simulink model "c00019M_harness"  (R2018a)
settings: Solver=ode3  StartTime=0.0  StopTime=10.0  RelTol=1e-3  EnableMultiTasking=on
undefined symbols (not defined in the file): b, DiscIntNeverNeededParam, J, K, L, PosMinimaW4, R, sigbuilder_block
(part 7 of 43)

== system c00019M_harness/M063 ==
  DW1 : Inport  OutMin=0  OutMax=4  OutDataTypeStr=int8
  P1W2 : Inport  Port=2  OutMin=0  OutMax=4  OutDataTypeStr=int8
  P3W4 : Inport  Port=3  OutMin=0  OutMax=4  OutDataTypeStr=int8
  O1 : Inport  Port=4  OutDataTypeStr=boolean
  O2 : Inport  Port=5  OutDataTypeStr=boolean
  O4 : Inport  Port=6  OutDataTypeStr=boolean
  LD : Inport  Port=7  OutDataTypeStr=boolean
  CW1C : Inport  Port=8  OutMin=0  OutMax=4  OutDataTypeStr=int8
  CW2C : Inport  Port=9  OutMin=0  OutMax=4  OutDataTypeStr=int8
  CW4C : Inport  Port=10  OutMin=0  OutMax=4  OutDataTypeStr=int8
  Cyber : Subsystem
  M : Memory
  M1 : Memory
  M3 : Memory
  Physical : Subsystem
  S1 : Subsystem
  S2 : Subsystem
  S4 : Subsystem
  W1Pos : Outport
  W2Pos : Outport  Port=2
  W4Pos : Outport  Port=3
  wires:
  Cyber/3(W4) -> Physical/3(InW4)
  Physical/3(W4) -> S4/1(PhyMeasure), W4Pos/1
  P3W4/1 -> Cyber/6(P3W4)
  S2/1(SensorOut) -> M1/1
  Physical/2(W2) -> S2/1(PhyMeasure), W2Pos/1
  DW1/1 -> Cyber/4(DW1)
  M/1 -> Cyber/1(PosW1)
  M1/1 -> Cyber/2(PosW2)
  S4/1(SensorOut) -> M3/1
  CW1C/1 -> Cyber/11(CW1C)
  P1W2/1 -> Cyber/5(P1W2)
  Cyber/2(W2) -> Physical/2(InW2)
  Cyber/1(W1) -> Physical/1(InW1)
  O1/1 -> Cyber/7(OW1)
  LD/1 -> Cyber/10(LD)
  O2/1 -> Cyber/8(OW2)
  O4/1 -> Cyber/9(OW4)
  Physical/1(W1) -> S1/1(PhyMeasure), W1Pos/1
  CW4C/1 -> Cyber/13(CW4C)
  CW2C/1 -> Cyber/12(CW2C)
  S1/1(SensorOut) -> M/1
  M3/1 -> Cyber/3(PosW4)

== system c00019M_harness/M064 ==
  DW1 : Inport  OutMin=0  OutMax=4  OutDataTypeStr=int8
  P1W2 : Inport  Port=2  OutMin=0  OutMax=4  OutDataTypeStr=int8
  P3W4 : Inport  Port=3  OutMin=0  OutMax=4  OutDataTypeStr=int8
  O1 : Inport  Port=4  OutDataTypeStr=boolean
  O2 : Inport  Port=5  OutDataTypeStr=boolean
  O4 : Inport  Port=6  OutDataTypeStr=boolean
  LD : Inport  Port=7  OutDataTypeStr=boolean
  CW1C : Inport  Port=8  OutMin=0  OutMax=4  OutDataTypeStr=int8
  CW2C : Inport  Port=9  OutMin=0  OutMax=4  OutDataTypeStr=int8
  CW4C : Inport  Port=10  OutMin=0  OutMax=4  OutDataTypeStr=int8
  Cyber : Subsystem
  M : Memory
  M1 : Memory
  M3 : Memory
  Physical : Subsystem
  S1 : Subsystem
  S2 : Subsystem
  S4 : Subsystem
  W1Pos : Outport
  W2Pos : Outport  Port=2
  W4Pos : Outport  Port=3
  wires:
  Cyber/3(W4) -> Physical/3(InW4)
  Physical/3(W4) -> S4/1(PhyMeasure), W4Pos/1
  P3W4/1 -> Cyber/6(P3W4)
  S2/1(SensorOut) -> M1/1
  Physical/2(W2) -> S2/1(PhyMeasure), W2Pos/1
  DW1/1 -> Cyber/4(DW1)
  M/1 -> Cyber/1(PosW1)
  M1/1 -> Cyber/2(PosW2)
  S4/1(SensorOut) -> M3/1
  CW1C/1 -> Cyber/11(CW1C)
  P1W2/1 -> Cyber/5(P1W2)
  Cyber/2(W2) -> Physical/2(InW2)
  Cyber/1(W1) -> Physical/1(InW1)
  O1/1 -> Cyber/7(OW1)
  LD/1 -> Cyber/10(LD)
  O2/1 -> Cyber/8(OW2)
  O4/1 -> Cyber/9(OW4)
  Physical/1(W1) -> S1/1(PhyMeasure), W1Pos/1
  CW4C/1 -> Cyber/13(CW4C)
  CW2C/1 -> Cyber/12(CW2C)
  S1/1(SensorOut) -> M/1
  M3/1 -> Cyber/3(PosW4)

== system c00019M_harness/M066 ==
  DW1 : Inport  OutMin=0  OutMax=4  OutDataTypeStr=int8
  P1W2 : Inport  Port=2  OutMin=0  OutMax=4  OutDataTypeStr=int8
  P3W4 : Inport  Port=3  OutMin=0  OutMax=4  OutDataTypeStr=int8
  O1 : Inport  Port=4  OutDataTypeStr=boolean
  O2 : Inport  Port=5  OutDataTypeStr=boolean
  O4 : Inport  Port=6  OutDataTypeStr=boolean
  LD : Inport  Port=7  OutDataTypeStr=boolean
  CW1C : Inport  Port=8  OutMin=0  OutMax=4  OutDataTypeStr=int8
  CW2C : Inport  Port=9  OutMin=0  OutMax=4  OutDataTypeStr=int8
  CW4C : Inport  Port=10  OutMin=0  OutMax=4  OutDataTypeStr=int8
  Cyber : Subsystem
  M : Memory
  M1 : Memory
  M3 : Memory
  Physical : Subsystem
  S1 : Subsystem
  S2 : Subsystem
  S4 : Subsystem
  W1Pos : Outport
  W2Pos : Outport  Port=2
  W4Pos : Outport  Port=3
  wires:
  Cyber/3(W4) -> Physical/3(InW4)
  Physical/3(W4) -> S4/1(PhyMeasure), W4Pos/1
  P3W4/1 -> Cyber/6(P3W4)
  S2/1(SensorOut) -> M1/1
  Physical/2(W2) -> S2/1(PhyMeasure), W2Pos/1
  DW1/1 -> Cyber/4(DW1)
  M/1 -> Cyber/1(PosW1)
  M1/1 -> Cyber/2(PosW2)
  S4/1(SensorOut) -> M3/1
  CW1C/1 -> Cyber/11(CW1C)
  P1W2/1 -> Cyber/5(P1W2)
  Cyber/2(W2) -> Physical/2(InW2)
  Cyber/1(W1) -> Physical/1(InW1)
  O1/1 -> Cyber/7(OW1)
  LD/1 -> Cyber/10(LD)
  O2/1 -> Cyber/8(OW2)
  O4/1 -> Cyber/9(OW4)
  Physical/1(W1) -> S1/1(PhyMeasure), W1Pos/1
  CW4C/1 -> Cyber/13(CW4C)
  CW2C/1 -> Cyber/12(CW2C)
  S1/1(SensorOut) -> M/1
  M3/1 -> Cyber/3(PosW4)

== system c00019M_harness/M067 ==
  DW1 : Inport  OutMin=0  OutMax=4  OutDataTypeStr=int8
  P1W2 : Inport  Port=2  OutMin=0  OutMax=4  OutDataTypeStr=int8
  P3W4 : Inport  Port=3  OutMin=0  OutMax=4  OutDataTypeStr=int8
  O1 : Inport  Port=4  OutDataTypeStr=boolean
  O2 : Inport  Port=5  OutDataTypeStr=boolean
  O4 : Inport  Port=6  OutDataTypeStr=boolean
  LD : Inport  Port=7  OutDataTypeStr=boolean
  CW1C : Inport  Port=8  OutMin=0  OutMax=4  OutDataTypeStr=int8
  CW2C : Inport  Port=9  OutMin=0  OutMax=4  OutDataTypeStr=int8
  CW4C : Inport  Port=10  OutMin=0  OutMax=4  OutDataTypeStr=int8
  Cyber : Subsystem
  M : Memory
  M1 : Memory
  M3 : Memory
  Physical : Subsystem
  S1 : Subsystem
  S2 : Subsystem
  S4 : Subsystem
  W1Pos : Outport
  W2Pos : Outport  Port=2
  W4Pos : Outport  Port=3
  wires:
  Cyber/3(W4) -> Physical/3(InW4)
  Physical/3(W4) -> S4/1(PhyMeasure), W4Pos/1
  P3W4/1 -> Cyber/6(P3W4)
  S2/1(SensorOut) -> M1/1
  Physical/2(W2) -> S2/1(PhyMeasure), W2Pos/1
  DW1/1 -> Cyber/4(DW1)
  M/1 -> Cyber/1(PosW1)
  M1/1 -> Cyber/2(PosW2)
  S4/1(SensorOut) -> M3/1
  CW1C/1 -> Cyber/11(CW1C)
  P1W2/1 -> Cyber/5(P1W2)
  Cyber/2(W2) -> Physical/2(InW2)
  Cyber/1(W1) -> Physical/1(InW1)
  O1/1 -> Cyber/7(OW1)
  LD/1 -> Cyber/10(LD)
  O2/1 -> Cyber/8(OW2)
  O4/1 -> Cyber/9(OW4)
  Physical/1(W1) -> S1/1(PhyMeasure), W1Pos/1
  CW4C/1 -> Cyber/13(CW4C)
  CW2C/1 -> Cyber/12(CW2C)
  S1/1(SensorOut) -> M/1
  M3/1 -> Cyber/3(PosW4)

== system c00019M_harness/M068 ==
  DW1 : Inport  OutMin=0  OutMax=4  OutDataTypeStr=int8
  P1W2 : Inport  Port=2  OutMin=0  OutMax=4  OutDataTypeStr=int8
  P3W4 : Inport  Port=3  OutMin=0  OutMax=4  OutDataTypeStr=int8
  O1 : Inport  Port=4  OutDataTypeStr=boolean
  O2 : Inport  Port=5  OutDataTypeStr=boolean
  O4 : Inport  Port=6  OutDataTypeStr=boolean
  LD : Inport  Port=7  OutDataTypeStr=boolean
  CW1C : Inport  Port=8  OutMin=0  OutMax=4  OutDataTypeStr=int8
  CW2C : Inport  Port=9  OutMin=0  OutMax=4  OutDataTypeStr=int8
  CW4C : Inport  Port=10  OutMin=0  OutMax=4  OutDataTypeStr=int8
  Cyber : Subsystem
  M : Memory
  M1 : Memory
  M3 : Memory
  Physical : Subsystem
  S1 : Subsystem
  S2 : Subsystem
  S4 : Subsystem
  W1Pos : Outport
  W2Pos : Outport  Port=2
  W4Pos : Outport  Port=3
  wires:
  Cyber/3(W4) -> Physical/3(InW4)
  Physical/3(W4) -> S4/1(PhyMeasure), W4Pos/1
  P3W4/1 -> Cyber/6(P3W4)
  S2/1(SensorOut) -> M1/1
  Physical/2(W2) -> S2/1(PhyMeasure), W2Pos/1
  DW1/1 -> Cyber/4(DW1)
  M/1 -> Cyber/1(PosW1)
  M1/1 -> Cyber/2(PosW2)
  S4/1(SensorOut) -> M3/1
  CW1C/1 -> Cyber/11(CW1C)
  P1W2/1 -> Cyber/5(P1W2)
  Cyber/2(W2) -> Physical/2(InW2)
  Cyber/1(W1) -> Physical/1(InW1)
  O1/1 -> Cyber/7(OW1)
  LD/1 -> Cyber/10(LD)
  O2/1 -> Cyber/8(OW2)
  O4/1 -> Cyber/9(OW4)
  Physical/1(W1) -> S1/1(PhyMeasure), W1Pos/1
  CW4C/1 -> Cyber/13(CW4C)
  CW2C/1 -> Cyber/12(CW2C)
  S1/1(SensorOut) -> M/1
  M3/1 -> Cyber/3(PosW4)

== system c00019M_harness/M070 ==
  DW1 : Inport  OutMin=0  OutMax=4  OutDataTypeStr=int8
  P1W2 : Inport  Port=2  OutMin=0  OutMax=4  OutDataTypeStr=int8
  P3W4 : Inport  Port=3  OutMin=0  OutMax=4  OutDataTypeStr=int8
  O1 : Inport  Port=4  OutDataTypeStr=boolean
  O2 : Inport  Port=5  OutDataTypeStr=boolean
  O4 : Inport  Port=6  OutDataTypeStr=boolean
  LD : Inport  Port=7  OutDataTypeStr=boolean
  CW1C : Inport  Port=8  OutMin=0  OutMax=4  OutDataTypeStr=int8
  CW2C : Inport  Port=9  OutMin=0  OutMax=4  OutDataTypeStr=int8
  CW4C : Inport  Port=10  OutMin=0  OutMax=4  OutDataTypeStr=int8
  Cyber : Subsystem
  M : Memory
  M1 : Memory
  M3 : Memory
  Physical : Subsystem
  S1 : Subsystem
  S2 : Subsystem
  S4 : Subsystem
  W1Pos : Outport
  W2Pos : Outport  Port=2
  W4Pos : Outport  Port=3
  wires:
  Cyber/3(W4) -> Physical/3(InW4)
  Physical/3(W4) -> S4/1(PhyMeasure), W4Pos/1
  P3W4/1 -> Cyber/6(P3W4)
  S2/1(SensorOut) -> M1/1
  Physical/2(W2) -> S2/1(PhyMeasure), W2Pos/1
  DW1/1 -> Cyber/4(DW1)
  M/1 -> Cyber/1(PosW1)
  M1/1 -> Cyber/2(PosW2)
  S4/1(SensorOut) -> M3/1
  CW1C/1 -> Cyber/11(CW1C)
  P1W2/1 -> Cyber/5(P1W2)
  Cyber/2(W2) -> Physical/2(InW2)
  Cyber/1(W1) -> Physical/1(InW1)
  O1/1 -> Cyber/7(OW1)
  LD/1 -> Cyber/10(LD)
  O2/1 -> Cyber/8(OW2)
  O4/1 -> Cyber/9(OW4)
  Physical/1(W1) -> S1/1(PhyMeasure), W1Pos/1
  CW4C/1 -> Cyber/13(CW4C)
  CW2C/1 -> Cyber/12(CW2C)
  S1/1(SensorOut) -> M/1
  M3/1 -> Cyber/3(PosW4)

== system c00019M_harness/M071 ==
  DW1 : Inport  OutMin=0  OutMax=4  OutDataTypeStr=int8
  P1W2 : Inport  Port=2  OutMin=0  OutMax=4  OutDataTypeStr=int8
  P3W4 : Inport  Port=3  OutMin=0  OutMax=4  OutDataTypeStr=int8
  O1 : Inport  Port=4  OutDataTypeStr=boolean
  O2 : Inport  Port=5  OutDataTypeStr=boolean
  O4 : Inport  Port=6  OutDataTypeStr=boolean
  LD : Inport  Port=7  OutDataTypeStr=boolean
  CW1C : Inport  Port=8  OutMin=0  OutMax=4  OutDataTypeStr=int8
  CW2C : Inport  Port=9  OutMin=0  OutMax=4  OutDataTypeStr=int8
  CW4C : Inport  Port=10  OutMin=0  OutMax=4  OutDataTypeStr=int8
  Cyber : Subsystem
  M : Memory
  M1 : Memory
  M3 : Memory
  Physical : Subsystem
  S1 : Subsystem
  S2 : Subsystem
  S4 : Subsystem
  W1Pos : Outport
  W2Pos : Outport  Port=2
  W4Pos : Outport  Port=3
  wires:
  Cyber/3(W4) -> Physical/3(InW4)
  Physical/3(W4) -> S4/1(PhyMeasure), W4Pos/1
  P3W4/1 -> Cyber/6(P3W4)
  S2/1(SensorOut) -> M1/1
  Physical/2(W2) -> S2/1(PhyMeasure), W2Pos/1
  DW1/1 -> Cyber/4(DW1)
  M/1 -> Cyber/1(PosW1)
  M1/1 -> Cyber/2(PosW2)
  S4/1(SensorOut) -> M3/1
  CW1C/1 -> Cyber/11(CW1C)
  P1W2/1 -> Cyber/5(P1W2)
  Cyber/2(W2) -> Physical/2(InW2)
  Cyber/1(W1) -> Physical/1(InW1)
  O1/1 -> Cyber/7(OW1)
  LD/1 -> Cyber/10(LD)
  O2/1 -> Cyber/8(OW2)
  O4/1 -> Cyber/9(OW4)
  Physical/1(W1) -> S1/1(PhyMeasure), W1Pos/1
  CW4C/1 -> Cyber/13(CW4C)
  CW2C/1 -> Cyber/12(CW2C)
  S1/1(SensorOut) -> M/1
  M3/1 -> Cyber/3(PosW4)

== system c00019M_harness/M072 ==
  DW1 : Inport  OutMin=0  OutMax=4  OutDataTypeStr=int8
  P1W2 : Inport  Port=2  OutMin=0  OutMax=4  OutDataTypeStr=int8
  P3W4 : Inport  Port=3  OutMin=0  OutMax=4  OutDataTypeStr=int8
  O1 : Inport  Port=4  OutDataTypeStr=boolean
  O2 : Inport  Port=5  OutDataTypeStr=boolean
  O4 : Inport  Port=6  OutDataTypeStr=boolean
  LD : Inport  Port=7  OutDataTypeStr=boolean
  CW1C : Inport  Port=8  OutMin=0  OutMax=4  OutDataTypeStr=int8
  CW2C : Inport  Port=9  OutMin=0  OutMax=4  OutDataTypeStr=int8
  CW4C : Inport  Port=10  OutMin=0  OutMax=4  OutDataTypeStr=int8
  Cyber : Subsystem
  M : Memory
  M1 : Memory
  M3 : Memory
  Physical : Subsystem
  S1 : Subsystem
  S2 : Subsystem
  S4 : Subsystem
  W1Pos : Outport
  W2Pos : Outport  Port=2
  W4Pos : Outport  Port=3
  wires:
  Cyber/3(W4) -> Physical/3(InW4)
  Physical/3(W4) -> S4/1(PhyMeasure), W4Pos/1
  P3W4/1 -> Cyber/6(P3W4)
  S2/1(SensorOut) -> M1/1
  Physical/2(W2) -> S2/1(PhyMeasure), W2Pos/1
  DW1/1 -> Cyber/4(DW1)
  M/1 -> Cyber/1(PosW1)
  M1/1 -> Cyber/2(PosW2)
  S4/1(SensorOut) -> M3/1
  CW1C/1 -> Cyber/11(CW1C)
  P1W2/1 -> Cyber/5(P1W2)
  Cyber/2(W2) -> Physical/2(InW2)
  Cyber/1(W1) -> Physical/1(InW1)
  O1/1 -> Cyber/7(OW1)
  LD/1 -> Cyber/10(LD)
  O2/1 -> Cyber/8(OW2)
  O4/1 -> Cyber/9(OW4)
  Physical/1(W1) -> S1/1(PhyMeasure), W1Pos/1
  CW4C/1 -> Cyber/13(CW4C)
  CW2C/1 -> Cyber/12(CW2C)
  S1/1(SensorOut) -> M/1
  M3/1 -> Cyber/3(PosW4)

== system c00019M_harness/M074 ==
  DW1 : Inport  OutMin=0  OutMax=4  OutDataTypeStr=int8
  P1W2 : Inport  Port=2  OutMin=0  OutMax=4  OutDataTypeStr=int8
  P3W4 : Inport  Port=3  OutMin=0  OutMax=4  OutDataTypeStr=int8
  O1 : Inport  Port=4  OutDataTypeStr=boolean
  O2 : Inport  Port=5  OutDataTypeStr=boolean
  O4 : Inport  Port=6  OutDataTypeStr=boolean
  LD : Inport  Port=7  OutDataTypeStr=boolean
  CW1C : Inport  Port=8  OutMin=0  OutMax=4  OutDataTypeStr=int8
  CW2C : Inport  Port=9  OutMin=0  OutMax=4  OutDataTypeStr=int8
  CW4C : Inport  Port=10  OutMin=0  OutMax=4  OutDataTypeStr=int8
  Cyber : Subsystem
  M : Memory
  M1 : Memory
  M3 : Memory
  Physical : Subsystem
  S1 : Subsystem
  S2 : Subsystem
  S4 : Subsystem
  W1Pos : Outport
  W2Pos : Outport  Port=2
  W4Pos : Outport  Port=3
  wires:
  Cyber/3(W4) -> Physical/3(InW4)
  Physical/3(W4) -> S4/1(PhyMeasure), W4Pos/1
  P3W4/1 -> Cyber/6(P3W4)
  S2/1(SensorOut) -> M1/1
  Physical/2(W2) -> S2/1(PhyMeasure), W2Pos/1
  DW1/1 -> Cyber/4(DW1)
  M/1 -> Cyber/1(PosW1)
  M1/1 -> Cyber/2(PosW2)
  S4/1(SensorOut) -> M3/1
  CW1C/1 -> Cyber/11(CW1C)
  P1W2/1 -> Cyber/5(P1W2)
  Cyber/2(W2) -> Physical/2(InW2)
  Cyber/1(W1) -> Physical/1(InW1)
  O1/1 -> Cyber/7(OW1)
  LD/1 -> Cyber/10(LD)
  O2/1 -> Cyber/8(OW2)
  O4/1 -> Cyber/9(OW4)
  Physical/1(W1) -> S1/1(PhyMeasure), W1Pos/1
  CW4C/1 -> Cyber/13(CW4C)
  CW2C/1 -> Cyber/12(CW2C)
  S1/1(SensorOut) -> M/1
  M3/1 -> Cyber/3(PosW4)

== system c00019M_harness/M075 ==
  DW1 : Inport  OutMin=0  OutMax=4  OutDataTypeStr=int8
  P1W2 : Inport  Port=2  OutMin=0  OutMax=4  OutDataTypeStr=int8
  P3W4 : Inport  Port=3  OutMin=0  OutMax=4  OutDataTypeStr=int8
  O1 : Inport  Port=4  OutDataTypeStr=boolean
  O2 : Inport  Port=5  OutDataTypeStr=boolean
  O4 : Inport  Port=6  OutDataTypeStr=boolean
  LD : Inport  Port=7  OutDataTypeStr=boolean
  CW1C : Inport  Port=8  OutMin=0  OutMax=4  OutDataTypeStr=int8
  CW2C : Inport  Port=9  OutMin=0  OutMax=4  OutDataTypeStr=int8
  CW4C : Inport  Port=10  OutMin=0  OutMax=4  OutDataTypeStr=int8
  Cyber : Subsystem
  M : Memory
  M1 : Memory
  M3 : Memory
  Physical : Subsystem
  S1 : Subsystem
  S2 : Subsystem
  S4 : Subsystem
  W1Pos : Outport
  W2Pos : Outport  Port=2
  W4Pos : Outport  Port=3
  wires:
  Cyber/3(W4) -> Physical/3(InW4)
  Physical/3(W4) -> S4/1(PhyMeasure), W4Pos/1
  P3W4/1 -> Cyber/6(P3W4)
  S2/1(SensorOut) -> M1/1
  Physical/2(W2) -> S2/1(PhyMeasure), W2Pos/1
  DW1/1 -> Cyber/4(DW1)
  M/1 -> Cyber/1(PosW1)
  M1/1 -> Cyber/2(PosW2)
  S4/1(SensorOut) -> M3/1
  CW1C/1 -> Cyber/11(CW1C)
  P1W2/1 -> Cyber/5(P1W2)
  Cyber/2(W2) -> Physical/2(InW2)
  Cyber/1(W1) -> Physical/1(InW1)
  O1/1 -> Cyber/7(OW1)
  LD/1 -> Cyber/10(LD)
  O2/1 -> Cyber/8(OW2)
  O4/1 -> Cyber/9(OW4)
  Physical/1(W1) -> S1/1(PhyMeasure), W1Pos/1
  CW4C/1 -> Cyber/13(CW4C)
  CW2C/1 -> Cyber/12(CW2C)
  S1/1(SensorOut) -> M/1
  M3/1 -> Cyber/3(PosW4)

== system c00019M_harness/M076 ==
  DW1 : Inport  OutMin=0  OutMax=4  OutDataTypeStr=int8
  P1W2 : Inport  Port=2  OutMin=0  OutMax=4  OutDataTypeStr=int8
  P3W4 : Inport  Port=3  OutMin=0  OutMax=4  OutDataTypeStr=int8
  O1 : Inport  Port=4  OutDataTypeStr=boolean
  O2 : Inport  Port=5  OutDataTypeStr=boolean
  O4 : Inport  Port=6  OutDataTypeStr=boolean
  LD : Inport  Port=7  OutDataTypeStr=boolean
  CW1C : Inport  Port=8  OutMin=0  OutMax=4  OutDataTypeStr=int8
  CW2C : Inport  Port=9  OutMin=0  OutMax=4  OutDataTypeStr=int8
  CW4C : Inport  Port=10  OutMin=0  OutMax=4  OutDataTypeStr=int8
  Cyber : Subsystem
  M : Memory
  M1 : Memory
  M3 : Memory
  Physical : Subsystem
  S1 : Subsystem
  S2 : Subsystem
  S4 : Subsystem
  W1Pos : Outport
  W2Pos : Outport  Port=2
  W4Pos : Outport  Port=3
  wires:
  Cyber/3(W4) -> Physical/3(InW4)
  Physical/3(W4) -> S4/1(PhyMeasure), W4Pos/1
  P3W4/1 -> Cyber/6(P3W4)
  S2/1(SensorOut) -> M1/1
  Physical/2(W2) -> S2/1(PhyMeasure), W2Pos/1
  DW1/1 -> Cyber/4(DW1)
  M/1 -> Cyber/1(PosW1)
  M1/1 -> Cyber/2(PosW2)
  S4/1(SensorOut) -> M3/1
  CW1C/1 -> Cyber/11(CW1C)
  P1W2/1 -> Cyber/5(P1W2)
  Cyber/2(W2) -> Physical/2(InW2)
  Cyber/1(W1) -> Physical/1(InW1)
  O1/1 -> Cyber/7(OW1)
  LD/1 -> Cyber/10(LD)
  O2/1 -> Cyber/8(OW2)
  O4/1 -> Cyber/9(OW4)
  Physical/1(W1) -> S1/1(PhyMeasure), W1Pos/1
  CW4C/1 -> Cyber/13(CW4C)
  CW2C/1 -> Cyber/12(CW2C)
  S1/1(SensorOut) -> M/1
  M3/1 -> Cyber/3(PosW4)

== system c00019M_harness/M078 ==
  DW1 : Inport  OutMin=0  OutMax=4  OutDataTypeStr=int8
  P1W2 : Inport  Port=2  OutMin=0  OutMax=4  OutDataTypeStr=int8
  P3W4 : Inport  Port=3  OutMin=0  OutMax=4  OutDataTypeStr=int8
  O1 : Inport  Port=4  OutDataTypeStr=boolean
  O2 : Inport  Port=5  OutDataTypeStr=boolean
  O4 : Inport  Port=6  OutDataTypeStr=boolean
  LD : Inport  Port=7  OutDataTypeStr=boolean
  CW1C : Inport  Port=8  OutMin=0  OutMax=4  OutDataTypeStr=int8
  CW2C : Inport  Port=9  OutMin=0  OutMax=4  OutDataTypeStr=int8
  CW4C : Inport  Port=10  OutMin=0  OutMax=4  OutDataTypeStr=int8
  Cyber : Subsystem
  M : Memory
  M1 : Memory
  M3 : Memory
  Physical : Subsystem
  S1 : Subsystem
  S2 : Subsystem
  S4 : Subsystem
  W1Pos : Outport
  W2Pos : Outport  Port=2
  W4Pos : Outport  Port=3
  wires:
  Cyber/3(W4) -> Physical/3(InW4)
  Physical/3(W4) -> S4/1(PhyMeasure), W4Pos/1
  P3W4/1 -> Cyber/6(P3W4)
  S2/1(SensorOut) -> M1/1
  Physical/2(W2) -> S2/1(PhyMeasure), W2Pos/1
  DW1/1 -> Cyber/4(DW1)
  M/1 -> Cyber/1(PosW1)
  M1/1 -> Cyber/2(PosW2)
  S4/1(SensorOut) -> M3/1
  CW1C/1 -> Cyber/11(CW1C)
  P1W2/1 -> Cyber/5(P1W2)
  Cyber/2(W2) -> Physical/2(InW2)
  Cyber/1(W1) -> Physical/1(InW1)
  O1/1 -> Cyber/7(OW1)
  LD/1 -> Cyber/10(LD)
  O2/1 -> Cyber/8(OW2)
  O4/1 -> Cyber/9(OW4)
  Physical/1(W1) -> S1/1(PhyMeasure), W1Pos/1
  CW4C/1 -> Cyber/13(CW4C)
  CW2C/1 -> Cyber/12(CW2C)
  S1/1(SensorOut) -> M/1
  M3/1 -> Cyber/3(PosW4)

== system c00019M_harness/M079 ==
  DW1 : Inport  OutMin=0  OutMax=4  OutDataTypeStr=int8
  P1W2 : Inport  Port=2  OutMin=0  OutMax=4  OutDataTypeStr=int8
  P3W4 : Inport  Port=3  OutMin=0  OutMax=4  OutDataTypeStr=int8
  O1 : Inport  Port=4  OutDataTypeStr=boolean
  O2 : Inport  Port=5  OutDataTypeStr=boolean
  O4 : Inport  Port=6  OutDataTypeStr=boolean
  LD : Inport  Port=7  OutDataTypeStr=boolean
  CW1C : Inport  Port=8  OutMin=0  OutMax=4  OutDataTypeStr=int8
  CW2C : Inport  Port=9  OutMin=0  OutMax=4  OutDataTypeStr=int8
  CW4C : Inport  Port=10  OutMin=0  OutMax=4  OutDataTypeStr=int8
  Cyber : Subsystem
  M : Memory
  M1 : Memory
  M3 : Memory
  Physical : Subsystem
  S1 : Subsystem
  S2 : Subsystem
  S4 : Subsystem
  W1Pos : Outport
  W2Pos : Outport  Port=2
  W4Pos : Outport  Port=3
  wires:
  Cyber/3(W4) -> Physical/3(InW4)
  Physical/3(W4) -> S4/1(PhyMeasure), W4Pos/1
  P3W4/1 -> Cyber/6(P3W4)
  S2/1(SensorOut) -> M1/1
  Physical/2(W2) -> S2/1(PhyMeasure), W2Pos/1
  DW1/1 -> Cyber/4(DW1)
  M/1 -> Cyber/1(PosW1)
  M1/1 -> Cyber/2(PosW2)
  S4/1(SensorOut) -> M3/1
  CW1C/1 -> Cyber/11(CW1C)
  P1W2/1 -> Cyber/5(P1W2)
  Cyber/2(W2) -> Physical/2(InW2)
  Cyber/1(W1) -> Physical/1(InW1)
  O1/1 -> Cyber/7(OW1)
  LD/1 -> Cyber/10(LD)
  O2/1 -> Cyber/8(OW2)
  O4/1 -> Cyber/9(OW4)
  Physical/1(W1) -> S1/1(PhyMeasure), W1Pos/1
  CW4C/1 -> Cyber/13(CW4C)
  CW2C/1 -> Cyber/12(CW2C)
  S1/1(SensorOut) -> M/1
  M3/1 -> Cyber/3(PosW4)

== system c00019M_harness/M080 ==
  DW1 : Inport  OutMin=0  OutMax=4  OutDataTypeStr=int8
  P1W2 : Inport  Port=2  OutMin=0  OutMax=4  OutDataTypeStr=int8
  P3W4 : Inport  Port=3  OutMin=0  OutMax=4  OutDataTypeStr=int8
  O1 : Inport  Port=4  OutDataTypeStr=boolean
  O2 : Inport  Port=5  OutDataTypeStr=boolean
  O4 : Inport  Port=6  OutDataTypeStr=boolean
  LD : Inport  Port=7  OutDataTypeStr=boolean
  CW1C : Inport  Port=8  OutMin=0  OutMax=4  OutDataTypeStr=int8
  CW2C : Inport  Port=9  OutMin=0  OutMax=4  OutDataTypeStr=int8
  CW4C : Inport  Port=10  OutMin=0  OutMax=4  OutDataTypeStr=int8
  Cyber : Subsystem
  M : Memory
  M1 : Memory
  M3 : Memory
  Physical : Subsystem
  S1 : Subsystem
  S2 : Subsystem
  S4 : Subsystem
  W1Pos : Outport
  W2Pos : Outport  Port=2
  W4Pos : Outport  Port=3
  wires:
  Cyber/3(W4) -> Physical/3(InW4)
  Physical/3(W4) -> S4/1(PhyMeasure), W4Pos/1
  P3W4/1 -> Cyber/6(P3W4)
  S2/1(SensorOut) -> M1/1
  Physical/2(W2) -> S2/1(PhyMeasure), W2Pos/1
  DW1/1 -> Cyber/4(DW1)
  M/1 -> Cyber/1(PosW1)
  M1/1 -> Cyber/2(PosW2)
  S4/1(SensorOut) -> M3/1
  CW1C/1 -> Cyber/11(CW1C)
  P1W2/1 -> Cyber/5(P1W2)
  Cyber/2(W2) -> Physical/2(InW2)
  Cyber/1(W1) -> Physical/1(InW1)
  O1/1 -> Cyber/7(OW1)
  LD/1 -> Cyber/10(LD)
  O2/1 -> Cyber/8(OW2)
  O4/1 -> Cyber/9(OW4)
  Physical/1(W1) -> S1/1(PhyMeasure), W1Pos/1
  CW4C/1 -> Cyber/13(CW4C)
  CW2C/1 -> Cyber/12(CW2C)
  S1/1(SensorOut) -> M/1
  M3/1 -> Cyber/3(PosW4)

== system c00019M_harness/M082 ==
  DW1 : Inport  OutMin=0  OutMax=4  OutDataTypeStr=int8
  P1W2 : Inport  Port=2  OutMin=0  OutMax=4  OutDataTypeStr=int8
  P3W4 : Inport  Port=3  OutMin=0  OutMax=4  OutDataTypeStr=int8
  O1 : Inport  Port=4  OutDataTypeStr=boolean
  O2 : Inport  Port=5  OutDataTypeStr=boolean
  O4 : Inport  Port=6  OutDataTypeStr=boolean
  LD : Inport  Port=7  OutDataTypeStr=boolean
  CW1C : Inport  Port=8  OutMin=0  OutMax=4  OutDataTypeStr=int8
  CW2C : Inport  Port=9  OutMin=0  OutMax=4  OutDataTypeStr=int8
  CW4C : Inport  Port=10  OutMin=0  OutMax=4  OutDataTypeStr=int8
  Cyber : Subsystem
  M : Memory
  M1 : Memory
  M3 : Memory
  Physical : Subsystem
  S1 : Subsystem
  S2 : Subsystem
  S4 : Subsystem
  W1Pos : Outport
  W2Pos : Outport  Port=2
  W4Pos : Outport  Port=3
  wires:
  Cyber/3(W4) -> Physical/3(InW4)
  Physical/3(W4) -> S4/1(PhyMeasure), W4Pos/1
  P3W4/1 -> Cyber/6(P3W4)
  S2/1(SensorOut) -> M1/1
  Physical/2(W2) -> S2/1(PhyMeasure), W2Pos/1
  DW1/1 -> Cyber/4(DW1)
  M/1 -> Cyber/1(PosW1)
  M1/1 -> Cyber/2(PosW2)
  S4/1(SensorOut) -> M3/1
  CW1C/1 -> Cyber/11(CW1C)
  P1W2/1 -> Cyber/5(P1W2)
  Cyber/2(W2) -> Physical/2(InW2)
  Cyber/1(W1) -> Physical/1(InW1)
  O1/1 -> Cyber/7(OW1)
  LD/1 -> Cyber/10(LD)
  O2/1 -> Cyber/8(OW2)
  O4/1 -> Cyber/9(OW4)
  Physical/1(W1) -> S1/1(PhyMeasure), W1Pos/1
  CW4C/1 -> Cyber/13(CW4C)
  CW2C/1 -> Cyber/12(CW2C)
  S1/1(SensorOut) -> M/1
  M3/1 -> Cyber/3(PosW4)

== system c00019M_harness/M083 ==
  DW1 : Inport  OutMin=0  OutMax=4  OutDataTypeStr=int8
  P1W2 : Inport  Port=2  OutMin=0  OutMax=4  OutDataTypeStr=int8
  P3W4 : Inport  Port=3  OutMin=0  OutMax=4  OutDataTypeStr=int8
  O1 : Inport  Port=4  OutDataTypeStr=boolean
  O2 : Inport  Port=5  OutDataTypeStr=boolean
  O4 : Inport  Port=6  OutDataTypeStr=boolean
  LD : Inport  Port=7  OutDataTypeStr=boolean
  CW1C : Inport  Port=8  OutMin=0  OutMax=4  OutDataTypeStr=int8
  CW2C : Inport  Port=9  OutMin=0  OutMax=4  OutDataTypeStr=int8
  CW4C : Inport  Port=10  OutMin=0  OutMax=4  OutDataTypeStr=int8
  Cyber : Subsystem
  M : Memory
  M1 : Memory
  M3 : Memory
  Physical : Subsystem
  S1 : Subsystem
  S2 : Subsystem
  S4 : Subsystem
  W1Pos : Outport
  W2Pos : Outport  Port=2
  W4Pos : Outport  Port=3
  wires:
  Cyber/3(W4) -> Physical/3(InW4)
  Physical/3(W4) -> S4/1(PhyMeasure), W4Pos/1
  P3W4/1 -> Cyber/6(P3W4)
  S2/1(SensorOut) -> M1/1
  Physical/2(W2) -> S2/1(PhyMeasure), W2Pos/1
  DW1/1 -> Cyber/4(DW1)
  M/1 -> Cyber/1(PosW1)
  M1/1 -> Cyber/2(PosW2)
  S4/1(SensorOut) -> M3/1
  CW1C/1 -> Cyber/11(CW1C)
  P1W2/1 -> Cyber/5(P1W2)
  Cyber/2(W2) -> Physical/2(InW2)
  Cyber/1(W1) -> Physical/1(InW1)
  O1/1 -> Cyber/7(OW1)
  LD/1 -> Cyber/10(LD)
  O2/1 -> Cyber/8(OW2)
  O4/1 -> Cyber/9(OW4)
  Physical/1(W1) -> S1/1(PhyMeasure), W1Pos/1
  CW4C/1 -> Cyber/13(CW4C)
  CW2C/1 -> Cyber/12(CW2C)
  S1/1(SensorOut) -> M/1
  M3/1 -> Cyber/3(PosW4)

== system c00019M_harness/M084 ==
  DW1 : Inport  OutMin=0  OutMax=4  OutDataTypeStr=int8
  P1W2 : Inport  Port=2  OutMin=0  OutMax=4  OutDataTypeStr=int8
  P3W4 : Inport  Port=3  OutMin=0  OutMax=4  OutDataTypeStr=int8
  O1 : Inport  Port=4  OutDataTypeStr=boolean
  O2 : Inport  Port=5  OutDataTypeStr=boolean
  O4 : Inport  Port=6  OutDataTypeStr=boolean
  LD : Inport  Port=7  OutDataTypeStr=boolean
  CW1C : Inport  Port=8  OutMin=0  OutMax=4  OutDataTypeStr=int8
  CW2C : Inport  Port=9  OutMin=0  OutMax=4  OutDataTypeStr=int8
  CW4C : Inport  Port=10  OutMin=0  OutMax=4  OutDataTypeStr=int8
  Cyber : Subsystem
  M : Memory
  M1 : Memory
  M3 : Memory
  Physical : Subsystem
  S1 : Subsystem
  S2 : Subsystem
  S4 : Subsystem
  W1Pos : Outport
  W2Pos : Outport  Port=2
  W4Pos : Outport  Port=3
  wires:
  Cyber/3(W4) -> Physical/3(InW4)
  Physical/3(W4) -> S4/1(PhyMeasure), W4Pos/1
  P3W4/1 -> Cyber/6(P3W4)
  S2/1(SensorOut) -> M1/1
  Physical/2(W2) -> S2/1(PhyMeasure), W2Pos/1
  DW1/1 -> Cyber/4(DW1)
  M/1 -> Cyber/1(PosW1)
  M1/1 -> Cyber/2(PosW2)
  S4/1(SensorOut) -> M3/1
  CW1C/1 -> Cyber/11(CW1C)
  P1W2/1 -> Cyber/5(P1W2)
  Cyber/2(W2) -> Physical/2(InW2)
  Cyber/1(W1) -> Physical/1(InW1)
  O1/1 -> Cyber/7(OW1)
  LD/1 -> Cyber/10(LD)
  O2/1 -> Cyber/8(OW2)
  O4/1 -> Cyber/9(OW4)
  Physical/1(W1) -> S1/1(PhyMeasure), W1Pos/1
  CW4C/1 -> Cyber/13(CW4C)
  CW2C/1 -> Cyber/12(CW2C)
  S1/1(SensorOut) -> M/1
  M3/1 -> Cyber/3(PosW4)

== system c00019M_harness/M086 ==
  DW1 : Inport  OutMin=0  OutMax=4  OutDataTypeStr=int8
  P1W2 : Inport  Port=2  OutMin=0  OutMax=4  OutDataTypeStr=int8
  P3W4 : Inport  Port=3  OutMin=0  OutMax=4  OutDataTypeStr=int8
  O1 : Inport  Port=4  OutDataTypeStr=boolean
  O2 : Inport  Port=5  OutDataTypeStr=boolean
  O4 : Inport  Port=6  OutDataTypeStr=boolean
  LD : Inport  Port=7  OutDataTypeStr=boolean
  CW1C : Inport  Port=8  OutMin=0  OutMax=4  OutDataTypeStr=int8
  CW2C : Inport  Port=9  OutMin=0  OutMax=4  OutDataTypeStr=int8
  CW4C : Inport  Port=10  OutMin=0  OutMax=4  OutDataTypeStr=int8
  Cyber : Subsystem
  M : Memory
  M1 : Memory
  M3 : Memory
  Physical : Subsystem
  S1 : Subsystem
  S2 : Subsystem
  S4 : Subsystem
  W1Pos : Outport
  W2Pos : Outport  Port=2
  W4Pos : Outport  Port=3
  wires:
  Cyber/3(W4) -> Physical/3(InW4)
  Physical/3(W4) -> S4/1(PhyMeasure), W4Pos/1
  P3W4/1 -> Cyber/6(P3W4)
  S2/1(SensorOut) -> M1/1
  Physical/2(W2) -> S2/1(PhyMeasure), W2Pos/1
  DW1/1 -> Cyber/4(DW1)
  M/1 -> Cyber/1(PosW1)
  M1/1 -> Cyber/2(PosW2)
  S4/1(SensorOut) -> M3/1
  CW1C/1 -> Cyber/11(CW1C)
  P1W2/1 -> Cyber/5(P1W2)
  Cyber/2(W2) -> Physical/2(InW2)
  Cyber/1(W1) -> Physical/1(InW1)
  O1/1 -> Cyber/7(OW1)
  LD/1 -> Cyber/10(LD)
  O2/1 -> Cyber/8(OW2)
  O4/1 -> Cyber/9(OW4)
  Physical/1(W1) -> S1/1(PhyMeasure), W1Pos/1
  CW4C/1 -> Cyber/13(CW4C)
  CW2C/1 -> Cyber/12(CW2C)
  S1/1(SensorOut) -> M/1
  M3/1 -> Cyber/3(PosW4)

== system c00019M_harness/M087 ==
  DW1 : Inport  OutMin=0  OutMax=4  OutDataTypeStr=int8
  P1W2 : Inport  Port=2  OutMin=0  OutMax=4  OutDataTypeStr=int8
  P3W4 : Inport  Port=3  OutMin=0  OutMax=4  OutDataTypeStr=int8
  O1 : Inport  Port=4  OutDataTypeStr=boolean
  O2 : Inport  Port=5  OutDataTypeStr=boolean
  O4 : Inport  Port=6  OutDataTypeStr=boolean
  LD : Inport  Port=7  OutDataTypeStr=boolean
  CW1C : Inport  Port=8  OutMin=0  OutMax=4  OutDataTypeStr=int8
  CW2C : Inport  Port=9  OutMin=0  OutMax=4  OutDataTypeStr=int8
  CW4C : Inport  Port=10  OutMin=0  OutMax=4  OutDataTypeStr=int8
  Cyber : Subsystem
  M : Memory
  M1 : Memory
  M3 : Memory
  Physical : Subsystem
  S1 : Subsystem
  S2 : Subsystem
  S4 : Subsystem
  W1Pos : Outport
  W2Pos : Outport  Port=2
  W4Pos : Outport  Port=3
  wires:
  Cyber/3(W4) -> Physical/3(InW4)
  Physical/3(W4) -> S4/1(PhyMeasure), W4Pos/1
  P3W4/1 -> Cyber/6(P3W4)
  S2/1(SensorOut) -> M1/1
  Physical/2(W2) -> S2/1(PhyMeasure), W2Pos/1
  DW1/1 -> Cyber/4(DW1)
  M/1 -> Cyber/1(PosW1)
  M1/1 -> Cyber/2(PosW2)
  S4/1(SensorOut) -> M3/1
  CW1C/1 -> Cyber/11(CW1C)
  P1W2/1 -> Cyber/5(P1W2)
  Cyber/2(W2) -> Physical/2(InW2)
  Cyber/1(W1) -> Physical/1(InW1)
  O1/1 -> Cyber/7(OW1)
  LD/1 -> Cyber/10(LD)
  O2/1 -> Cyber/8(OW2)
  O4/1 -> Cyber/9(OW4)
  Physical/1(W1) -> S1/1(PhyMeasure), W1Pos/1
  CW4C/1 -> Cyber/13(CW4C)
  CW2C/1 -> Cyber/12(CW2C)
  S1/1(SensorOut) -> M/1
  M3/1 -> Cyber/3(PosW4)

== system c00019M_harness/M088 ==
  DW1 : Inport  OutMin=0  OutMax=4  OutDataTypeStr=int8
  P1W2 : Inport  Port=2  OutMin=0  OutMax=4  OutDataTypeStr=int8
  P3W4 : Inport  Port=3  OutMin=0  OutMax=4  OutDataTypeStr=int8
  O1 : Inport  Port=4  OutDataTypeStr=boolean
  O2 : Inport  Port=5  OutDataTypeStr=boolean
  O4 : Inport  Port=6  OutDataTypeStr=boolean
  LD : Inport  Port=7  OutDataTypeStr=boolean
  CW1C : Inport  Port=8  OutMin=0  OutMax=4  OutDataTypeStr=int8
  CW2C : Inport  Port=9  OutMin=0  OutMax=4  OutDataTypeStr=int8
  CW4C : Inport  Port=10  OutMin=0  OutMax=4  OutDataTypeStr=int8
  Cyber : Subsystem
  M : Memory
  M1 : Memory
  M3 : Memory
  Physical : Subsystem
  S1 : Subsystem
  S2 : Subsystem
  S4 : Subsystem
  W1Pos : Outport
  W2Pos : Outport  Port=2
  W4Pos : Outport  Port=3
  wires:
  Cyber/3(W4) -> Physical/3(InW4)
  Physical/3(W4) -> S4/1(PhyMeasure), W4Pos/1
  P3W4/1 -> Cyber/6(P3W4)
  S2/1(SensorOut) -> M1/1
  Physical/2(W2) -> S2/1(PhyMeasure), W2Pos/1
  DW1/1 -> Cyber/4(DW1)
  M/1 -> Cyber/1(PosW1)
  M1/1 -> Cyber/2(PosW2)
  S4/1(SensorOut) -> M3/1
  CW1C/1 -> Cyber/11(CW1C)
  P1W2/1 -> Cyber/5(P1W2)
  Cyber/2(W2) -> Physical/2(InW2)
  Cyber/1(W1) -> Physical/1(InW1)
  O1/1 -> Cyber/7(OW1)
  LD/1 -> Cyber/10(LD)
  O2/1 -> Cyber/8(OW2)
  O4/1 -> Cyber/9(OW4)
  Physical/1(W1) -> S1/1(PhyMeasure), W1Pos/1
  CW4C/1 -> Cyber/13(CW4C)
  CW2C/1 -> Cyber/12(CW2C)
  S1/1(SensorOut) -> M/1
  M3/1 -> Cyber/3(PosW4)

== system c00019M_harness/M090 ==
  DW1 : Inport  OutMin=0  OutMax=4  OutDataTypeStr=int8
  P1W2 : Inport  Port=2  OutMin=0  OutMax=4  OutDataTypeStr=int8
  P3W4 : Inport  Port=3  OutMin=0  OutMax=4  OutDataTypeStr=int8
  O1 : Inport  Port=4  OutDataTypeStr=boolean
  O2 : Inport  Port=5  OutDataTypeStr=boolean
  O4 : Inport  Port=6  OutDataTypeStr=boolean
  LD : Inport  Port=7  OutDataTypeStr=boolean
  CW1C : Inport  Port=8  OutMin=0  OutMax=4  OutDataTypeStr=int8
  CW2C : Inport  Port=9  OutMin=0  OutMax=4  OutDataTypeStr=int8
  CW4C : Inport  Port=10  OutMin=0  OutMax=4  OutDataTypeStr=int8
  Cyber : Subsystem
  M : Memory
  M1 : Memory
  M3 : Memory
  Physical : Subsystem
  S1 : Subsystem
  S2 : Subsystem
  S4 : Subsystem
  W1Pos : Outport
  W2Pos : Outport  Port=2
  W4Pos : Outport  Port=3
  wires:
  Cyber/3(W4) -> Physical/3(InW4)
  Physical/3(W4) -> S4/1(PhyMeasure), W4Pos/1
  P3W4/1 -> Cyber/6(P3W4)
  S2/1(SensorOut) -> M1/1
  Physical/2(W2) -> S2/1(PhyMeasure), W2Pos/1
  DW1/1 -> Cyber/4(DW1)
  M/1 -> Cyber/1(PosW1)
  M1/1 -> Cyber/2(PosW2)
  S4/1(SensorOut) -> M3/1
  CW1C/1 -> Cyber/11(CW1C)
  P1W2/1 -> Cyber/5(P1W2)
  Cyber/2(W2) -> Physical/2(InW2)
  Cyber/1(W1) -> Physical/1(InW1)
  O1/1 -> Cyber/7(OW1)
  LD/1 -> Cyber/10(LD)
  O2/1 -> Cyber/8(OW2)
  O4/1 -> Cyber/9(OW4)
  Physical/1(W1) -> S1/1(PhyMeasure), W1Pos/1
  CW4C/1 -> Cyber/13(CW4C)
  CW2C/1 -> Cyber/12(CW2C)
  S1/1(SensorOut) -> M/1
  M3/1 -> Cyber/3(PosW4)

== system c00019M_harness/M091 ==
  DW1 : Inport  OutMin=0  OutMax=4  OutDataTypeStr=int8
  P1W2 : Inport  Port=2  OutMin=0  OutMax=4  OutDataTypeStr=int8
  P3W4 : Inport  Port=3  OutMin=0  OutMax=4  OutDataTypeStr=int8
  O1 : Inport  Port=4  OutDataTypeStr=boolean
  O2 : Inport  Port=5  OutDataTypeStr=boolean
  O4 : Inport  Port=6  OutDataTypeStr=boolean
  LD : Inport  Port=7  OutDataTypeStr=boolean
  CW1C : Inport  Port=8  OutMin=0  OutMax=4  OutDataTypeStr=int8
  CW2C : Inport  Port=9  OutMin=0  OutMax=4  OutDataTypeStr=int8
  CW4C : Inport  Port=10  OutMin=0  OutMax=4  OutDataTypeStr=int8
  Cyber : Subsystem
  M : Memory
  M1 : Memory
  M3 : Memory
  Physical : Subsystem
  S1 : Subsystem
  S2 : Subsystem
  S4 : Subsystem
  W1Pos : Outport
  W2Pos : Outport  Port=2
  W4Pos : Outport  Port=3
  wires:
  Cyber/3(W4) -> Physical/3(InW4)
  Physical/3(W4) -> S4/1(PhyMeasure), W4Pos/1
  P3W4/1 -> Cyber/6(P3W4)
  S2/1(SensorOut) -> M1/1
  Physical/2(W2) -> S2/1(PhyMeasure), W2Pos/1
  DW1/1 -> Cyber/4(DW1)
  M/1 -> Cyber/1(PosW1)
  M1/1 -> Cyber/2(PosW2)
  S4/1(SensorOut) -> M3/1
  CW1C/1 -> Cyber/11(CW1C)
  P1W2/1 -> Cyber/5(P1W2)
  Cyber/2(W2) -> Physical/2(InW2)
  Cyber/1(W1) -> Physical/1(InW1)
  O1/1 -> Cyber/7(OW1)
  LD/1 -> Cyber/10(LD)
  O2/1 -> Cyber/8(OW2)
  O4/1 -> Cyber/9(OW4)
  Physical/1(W1) -> S1/1(PhyMeasure), W1Pos/1
  CW4C/1 -> Cyber/13(CW4C)
  CW2C/1 -> Cyber/12(CW2C)
  S1/1(SensorOut) -> M/1
  M3/1 -> Cyber/3(PosW4)

== system c00019M_harness/M092 ==
  DW1 : Inport  OutMin=0  OutMax=4  OutDataTypeStr=int8
  P1W2 : Inport  Port=2  OutMin=0  OutMax=4  OutDataTypeStr=int8
  P3W4 : Inport  Port=3  OutMin=0  OutMax=4  OutDataTypeStr=int8
  O1 : Inport  Port=4  OutDataTypeStr=boolean
  O2 : Inport  Port=5  OutDataTypeStr=boolean
  O4 : Inport  Port=6  OutDataTypeStr=boolean
  LD : Inport  Port=7  OutDataTypeStr=boolean
  CW1C : Inport  Port=8  OutMin=0  OutMax=4  OutDataTypeStr=int8
  CW2C : Inport  Port=9  OutMin=0  OutMax=4  OutDataTypeStr=int8
  CW4C : Inport  Port=10  OutMin=0  OutMax=4  OutDataTypeStr=int8
  Cyber : Subsystem
  M : Memory
  M1 : Memory
  M3 : Memory
  Physical : Subsystem
  S1 : Subsystem
  S2 : Subsystem
  S4 : Subsystem
  W1Pos : Outport
  W2Pos : Outport  Port=2
  W4Pos : Outport  Port=3
  wires:
  Cyber/3(W4) -> Physical/3(InW4)
  Physical/3(W4) -> S4/1(PhyMeasure), W4Pos/1
  P3W4/1 -> Cyber/6(P3W4)
  S2/1(SensorOut) -> M1/1
  Physical/2(W2) -> S2/1(PhyMeasure), W2Pos/1
  DW1/1 -> Cyber/4(DW1)
  M/1 -> Cyber/1(PosW1)
  M1/1 -> Cyber/2(PosW2)
  S4/1(SensorOut) -> M3/1
  CW1C/1 -> Cyber/11(CW1C)
  P1W2/1 -> Cyber/5(P1W2)
  Cyber/2(W2) -> Physical/2(InW2)
  Cyber/1(W1) -> Physical/1(InW1)
  O1/1 -> Cyber/7(OW1)
  LD/1 -> Cyber/10(LD)
  O2/1 -> Cyber/8(OW2)
  O4/1 -> Cyber/9(OW4)
  Physical/1(W1) -> S1/1(PhyMeasure), W1Pos/1
  CW4C/1 -> Cyber/13(CW4C)
  CW2C/1 -> Cyber/12(CW2C)
  S1/1(SensorOut) -> M/1
  M3/1 -> Cyber/3(PosW4)

== system c00019M_harness/M094 ==
  DW1 : Inport  OutMin=0  OutMax=4  OutDataTypeStr=int8
  P1W2 : Inport  Port=2  OutMin=0  OutMax=4  OutDataTypeStr=int8
  P3W4 : Inport  Port=3  OutMin=0  OutMax=4  OutDataTypeStr=int8
  O1 : Inport  Port=4  OutDataTypeStr=boolean
  O2 : Inport  Port=5  OutDataTypeStr=boolean
  O4 : Inport  Port=6  OutDataTypeStr=boolean
  LD : Inport  Port=7  OutDataTypeStr=boolean
  CW1C : Inport  Port=8  OutMin=0  OutMax=4  OutDataTypeStr=int8
  CW2C : Inport  Port=9  OutMin=0  OutMax=4  OutDataTypeStr=int8
  CW4C : Inport  Port=10  OutMin=0  OutMax=4  OutDataTypeStr=int8
  Cyber : Subsystem
  M : Memory
  M1 : Memory
  M3 : Memory
  Physical : Subsystem
  S1 : Subsystem
  S2 : Subsystem
  S4 : Subsystem
  W1Pos : Outport
  W2Pos : Outport  Port=2
  W4Pos : Outport  Port=3
  wires:
  Cyber/3(W4) -> Physical/3(InW4)
  Physical/3(W4) -> S4/1(PhyMeasure), W4Pos/1
  P3W4/1 -> Cyber/6(P3W4)
  S2/1(SensorOut) -> M1/1
  Physical/2(W2) -> S2/1(PhyMeasure), W2Pos/1
  DW1/1 -> Cyber/4(DW1)
  M/1 -> Cyber/1(PosW1)
  M1/1 -> Cyber/2(PosW2)
  S4/1(SensorOut) -> M3/1
  CW1C/1 -> Cyber/11(CW1C)
  P1W2/1 -> Cyber/5(P1W2)
  Cyber/2(W2) -> Physical/2(InW2)
  Cyber/1(W1) -> Physical/1(InW1)
  O1/1 -> Cyber/7(OW1)
  LD/1 -> Cyber/10(LD)
  O2/1 -> Cyber/8(OW2)
  O4/1 -> Cyber/9(OW4)
  Physical/1(W1) -> S1/1(PhyMeasure), W1Pos/1
  CW4C/1 -> Cyber/13(CW4C)
  CW2C/1 -> Cyber/12(CW2C)
  S1/1(SensorOut) -> M/1
  M3/1 -> Cyber/3(PosW4)

== system c00019M_harness/M095 ==
  DW1 : Inport  OutMin=0  OutMax=4  OutDataTypeStr=int8
  P1W2 : Inport  Port=2  OutMin=0  OutMax=4  OutDataTypeStr=int8
  P3W4 : Inport  Port=3  OutMin=0  OutMax=4  OutDataTypeStr=int8
  O1 : Inport  Port=4  OutDataTypeStr=boolean
  O2 : Inport  Port=5  OutDataTypeStr=boolean
  O4 : Inport  Port=6  OutDataTypeStr=boolean
  LD : Inport  Port=7  OutDataTypeStr=boolean
  CW1C : Inport  Port=8  OutMin=0  OutMax=4  OutDataTypeStr=int8
  CW2C : Inport  Port=9  OutMin=0  OutMax=4  OutDataTypeStr=int8
  CW4C : Inport  Port=10  OutMin=0  OutMax=4  OutDataTypeStr=int8
  Cyber : Subsystem
  M : Memory
  M1 : Memory
  M3 : Memory
  Physical : Subsystem
  S1 : Subsystem
  S2 : Subsystem
  S4 : Subsystem
  W1Pos : Outport
  W2Pos : Outport  Port=2
  W4Pos : Outport  Port=3
  wires:
  Cyber/3(W4) -> Physical/3(InW4)
  Physical/3(W4) -> S4/1(PhyMeasure), W4Pos/1
  P3W4/1 -> Cyber/6(P3W4)
  S2/1(SensorOut) -> M1/1
  Physical/2(W2) -> S2/1(PhyMeasure), W2Pos/1
  DW1/1 -> Cyber/4(DW1)
  M/1 -> Cyber/1(PosW1)
  M1/1 -> Cyber/2(PosW2)
  S4/1(SensorOut) -> M3/1
  CW1C/1 -> Cyber/11(CW1C)
  P1W2/1 -> Cyber/5(P1W2)
  Cyber/2(W2) -> Physical/2(InW2)
  Cyber/1(W1) -> Physical/1(InW1)
  O1/1 -> Cyber/7(OW1)
  LD/1 -> Cyber/10(LD)
  O2/1 -> Cyber/8(OW2)
  O4/1 -> Cyber/9(OW4)
  Physical/1(W1) -> S1/1(PhyMeasure), W1Pos/1
  CW4C/1 -> Cyber/13(CW4C)
  CW2C/1 -> Cyber/12(CW2C)
  S1/1(SensorOut) -> M/1
  M3/1 -> Cyber/3(PosW4)

== system c00019M_harness/M096 ==
  DW1 : Inport  OutMin=0  OutMax=4  OutDataTypeStr=int8
  P1W2 : Inport  Port=2  OutMin=0  OutMax=4  OutDataTypeStr=int8
  P3W4 : Inport  Port=3  OutMin=0  OutMax=4  OutDataTypeStr=int8
  O1 : Inport  Port=4  OutDataTypeStr=boolean
  O2 : Inport  Port=5  OutDataTypeStr=boolean
  O4 : Inport  Port=6  OutDataTypeStr=boolean
  LD : Inport  Port=7  OutDataTypeStr=boolean
  CW1C : Inport  Port=8  OutMin=0  OutMax=4  OutDataTypeStr=int8
  CW2C : Inport  Port=9  OutMin=0  OutMax=4  OutDataTypeStr=int8
  CW4C : Inport  Port=10  OutMin=0  OutMax=4  OutDataTypeStr=int8
  Cyber : Subsystem
  M : Memory
  M1 : Memory
  M3 : Memory
  Physical : Subsystem
  S1 : Subsystem
  S2 : Subsystem
  S4 : Subsystem
  W1Pos : Outport
  W2Pos : Outport  Port=2
  W4Pos : Outport  Port=3
  wires:
  Cyber/3(W4) -> Physical/3(InW4)
  Physical/3(W4) -> S4/1(PhyMeasure), W4Pos/1
  P3W4/1 -> Cyber/6(P3W4)
  S2/1(SensorOut) -> M1/1
  Physical/2(W2) -> S2/1(PhyMeasure), W2Pos/1
  DW1/1 -> Cyber/4(DW1)
  M/1 -> Cyber/1(PosW1)
  M1/1 -> Cyber/2(PosW2)
  S4/1(SensorOut) -> M3/1
  CW1C/1 -> Cyber/11(CW1C)
  P1W2/1 -> Cyber/5(P1W2)
  Cyber/2(W2) -> Physical/2(InW2)
  Cyber/1(W1) -> Physical/1(InW1)
  O1/1 -> Cyber/7(OW1)
  LD/1 -> Cyber/10(LD)
  O2/1 -> Cyber/8(OW2)
  O4/1 -> Cyber/9(OW4)
  Physical/1(W1) -> S1/1(PhyMeasure), W1Pos/1
  CW4C/1 -> Cyber/13(CW4C)
  CW2C/1 -> Cyber/12(CW2C)
  S1/1(SensorOut) -> M/1
  M3/1 -> Cyber/3(PosW4)

== system c00019M_harness/M098 ==
  DW1 : Inport  OutMin=0  OutMax=4  OutDataTypeStr=int8
  P1W2 : Inport  Port=2  OutMin=0  OutMax=4  OutDataTypeStr=int8
  P3W4 : Inport  Port=3  OutMin=0  OutMax=4  OutDataTypeStr=int8
  O1 : Inport  Port=4  OutDataTypeStr=boolean
  O2 : Inport  Port=5  OutDataTypeStr=boolean
  O4 : Inport  Port=6  OutDataTypeStr=boolean
  LD : Inport  Port=7  OutDataTypeStr=boolean
  CW1C : Inport  Port=8  OutMin=0  OutMax=4  OutDataTypeStr=int8
  CW2C : Inport  Port=9  OutMin=0  OutMax=4  OutDataTypeStr=int8
  CW4C : Inport  Port=10  OutMin=0  OutMax=4  OutDataTypeStr=int8
  Cyber : Subsystem
  M : Memory
  M1 : Memory
  M3 : Memory
  Physical : Subsystem
  S1 : Subsystem
  S2 : Subsystem
  S4 : Subsystem
  W1Pos : Outport
  W2Pos : Outport  Port=2
  W4Pos : Outport  Port=3
  wires:
  Cyber/3(W4) -> Physical/3(InW4)
  Physical/3(W4) -> S4/1(PhyMeasure), W4Pos/1
  P3W4/1 -> Cyber/6(P3W4)
  S2/1(SensorOut) -> M1/1
  Physical/2(W2) -> S2/1(PhyMeasure), W2Pos/1
  DW1/1 -> Cyber/4(DW1)
  M/1 -> Cyber/1(PosW1)
  M1/1 -> Cyber/2(PosW2)
  S4/1(SensorOut) -> M3/1
  CW1C/1 -> Cyber/11(CW1C)
  P1W2/1 -> Cyber/5(P1W2)
  Cyber/2(W2) -> Physical/2(InW2)
  Cyber/1(W1) -> Physical/1(InW1)
  O1/1 -> Cyber/7(OW1)
  LD/1 -> Cyber/10(LD)
  O2/1 -> Cyber/8(OW2)
  O4/1 -> Cyber/9(OW4)
  Physical/1(W1) -> S1/1(PhyMeasure), W1Pos/1
  CW4C/1 -> Cyber/13(CW4C)
  CW2C/1 -> Cyber/12(CW2C)
  S1/1(SensorOut) -> M/1
  M3/1 -> Cyber/3(PosW4)

== system c00019M_harness/M099 ==
  DW1 : Inport  OutMin=0  OutMax=4  OutDataTypeStr=int8
  P1W2 : Inport  Port=2  OutMin=0  OutMax=4  OutDataTypeStr=int8
  P3W4 : Inport  Port=3  OutMin=0  OutMax=4  OutDataTypeStr=int8
  O1 : Inport  Port=4  OutDataTypeStr=boolean
  O2 : Inport  Port=5  OutDataTypeStr=boolean
  O4 : Inport  Port=6  OutDataTypeStr=boolean
  LD : Inport  Port=7  OutDataTypeStr=boolean
  CW1C : Inport  Port=8  OutMin=0  OutMax=4  OutDataTypeStr=int8
  CW2C : Inport  Port=9  OutMin=0  OutMax=4  OutDataTypeStr=int8
  CW4C : Inport  Port=10  OutMin=0  OutMax=4  OutDataTypeStr=int8
  Cyber : Subsystem
  M : Memory
  M1 : Memory
  M3 : Memory
  Physical : Subsystem
  S1 : Subsystem
  S2 : Subsystem
  S4 : Subsystem
  W1Pos : Outport
  W2Pos : Outport  Port=2
  W4Pos : Outport  Port=3
  wires:
  Cyber/3(W4) -> Physical/3(InW4)
  Physical/3(W4) -> S4/1(PhyMeasure), W4Pos/1
  P3W4/1 -> Cyber/6(P3W4)
  S2/1(SensorOut) -> M1/1
  Physical/2(W2) -> S2/1(PhyMeasure), W2Pos/1
  DW1/1 -> Cyber/4(DW1)
  M/1 -> Cyber/1(PosW1)
  M1/1 -> Cyber/2(PosW2)
  S4/1(SensorOut) -> M3/1
  CW1C/1 -> Cyber/11(CW1C)
  P1W2/1 -> Cyber/5(P1W2)
  Cyber/2(W2) -> Physical/2(InW2)
  Cyber/1(W1) -> Physical/1(InW1)
  O1/1 -> Cyber/7(OW1)
  LD/1 -> Cyber/10(LD)
  O2/1 -> Cyber/8(OW2)
  O4/1 -> Cyber/9(OW4)
  Physical/1(W1) -> S1/1(PhyMeasure), W1Pos/1
  CW4C/1 -> Cyber/13(CW4C)
  CW2C/1 -> Cyber/12(CW2C)
  S1/1(SensorOut) -> M/1
  M3/1 -> Cyber/3(PosW4)

== system c00019M_harness/M100 ==
  DW1 : Inport  OutMin=0  OutMax=4  OutDataTypeStr=int8
  P1W2 : Inport  Port=2  OutMin=0  OutMax=4  OutDataTypeStr=int8
  P3W4 : Inport  Port=3  OutMin=0  OutMax=4  OutDataTypeStr=int8
  O1 : Inport  Port=4  OutDataTypeStr=boolean
  O2 : Inport  Port=5  OutDataTypeStr=boolean
  O4 : Inport  Port=6  OutDataTypeStr=boolean
  LD : Inport  Port=7  OutDataTypeStr=boolean
  CW1C : Inport  Port=8  OutMin=0  OutMax=4  OutDataTypeStr=int8
  CW2C : Inport  Port=9  OutMin=0  OutMax=4  OutDataTypeStr=int8
  CW4C : Inport  Port=10  OutMin=0  OutMax=4  OutDataTypeStr=int8
  Cyber : Subsystem
  M : Memory
  M1 : Memory
  M3 : Memory
  Physical : Subsystem
  S1 : Subsystem
  S2 : Subsystem
  S4 : Subsystem
  W1Pos : Outport
  W2Pos : Outport  Port=2
  W4Pos : Outport  Port=3
  wires:
  Cyber/3(W4) -> Physical/3(InW4)
  Physical/3(W4) -> S4/1(PhyMeasure), W4Pos/1
  P3W4/1 -> Cyber/6(P3W4)
  S2/1(SensorOut) -> M1/1
  Physical/2(W2) -> S2/1(PhyMeasure), W2Pos/1
  DW1/1 -> Cyber/4(DW1)
  M/1 -> Cyber/1(PosW1)
  M1/1 -> Cyber/2(PosW2)
  S4/1(SensorOut) -> M3/1
  CW1C/1 -> Cyber/11(CW1C)
  P1W2/1 -> Cyber/5(P1W2)
  Cyber/2(W2) -> Physical/2(InW2)
  Cyber/1(W1) -> Physical/1(InW1)
  O1/1 -> Cyber/7(OW1)
  LD/1 -> Cyber/10(LD)
  O2/1 -> Cyber/8(OW2)
  O4/1 -> Cyber/9(OW4)
  Physical/1(W1) -> S1/1(PhyMeasure), W1Pos/1
  CW4C/1 -> Cyber/13(CW4C)
  CW2C/1 -> Cyber/12(CW2C)
  S1/1(SensorOut) -> M/1
  M3/1 -> Cyber/3(PosW4)

== system c00019M_harness/M102 ==
  DW1 : Inport  OutMin=0  OutMax=4  OutDataTypeStr=int8
  P1W2 : Inport  Port=2  OutMin=0  OutMax=4  OutDataTypeStr=int8
  P3W4 : Inport  Port=3  OutMin=0  OutMax=4  OutDataTypeStr=int8
  O1 : Inport  Port=4  OutDataTypeStr=boolean
  O2 : Inport  Port=5  OutDataTypeStr=boolean
  O4 : Inport  Port=6  OutDataTypeStr=boolean
  LD : Inport  Port=7  OutDataTypeStr=boolean
  CW1C : Inport  Port=8  OutMin=0  OutMax=4  OutDataTypeStr=int8
  CW2C : Inport  Port=9  OutMin=0  OutMax=4  OutDataTypeStr=int8
  CW4C : Inport  Port=10  OutMin=0  OutMax=4  OutDataTypeStr=int8
  Cyber : Subsystem
  M : Memory
  M1 : Memory
  M3 : Memory
  Physical : Subsystem
  S1 : Subsystem
  S2 : Subsystem
  S4 : Subsystem
  W1Pos : Outport
  W2Pos : Outport  Port=2
  W4Pos : Outport  Port=3
  wires:
  Cyber/3(W4) -> Physical/3(InW4)
  Physical/3(W4) -> S4/1(PhyMeasure), W4Pos/1
  P3W4/1 -> Cyber/6(P3W4)
  S2/1(SensorOut) -> M1/1
  Physical/2(W2) -> S2/1(PhyMeasure), W2Pos/1
  DW1/1 -> Cyber/4(DW1)
  M/1 -> Cyber/1(PosW1)
  M1/1 -> Cyber/2(PosW2)
  S4/1(SensorOut) -> M3/1
  CW1C/1 -> Cyber/11(CW1C)
  P1W2/1 -> Cyber/5(P1W2)
  Cyber/2(W2) -> Physical/2(InW2)
  Cyber/1(W1) -> Physical/1(InW1)
  O1/1 -> Cyber/7(OW1)
  LD/1 -> Cyber/10(LD)
  O2/1 -> Cyber/8(OW2)
  O4/1 -> Cyber/9(OW4)
  Physical/1(W1) -> S1/1(PhyMeasure), W1Pos/1
  CW4C/1 -> Cyber/13(CW4C)
  CW2C/1 -> Cyber/12(CW2C)
  S1/1(SensorOut) -> M/1
  M3/1 -> Cyber/3(PosW4)

== system c00019M_harness/M103 ==
  DW1 : Inport  OutMin=0  OutMax=4  OutDataTypeStr=int8
  P1W2 : Inport  Port=2  OutMin=0  OutMax=4  OutDataTypeStr=int8
  P3W4 : Inport  Port=3  OutMin=0  OutMax=4  OutDataTypeStr=int8
  O1 : Inport  Port=4  OutDataTypeStr=boolean
  O2 : Inport  Port=5  OutDataTypeStr=boolean
  O4 : Inport  Port=6  OutDataTypeStr=boolean
  LD : Inport  Port=7  OutDataTypeStr=boolean
  CW1C : Inport  Port=8  OutMin=0  OutMax=4  OutDataTypeStr=int8
  CW2C : Inport  Port=9  OutMin=0  OutMax=4  OutDataTypeStr=int8
  CW4C : Inport  Port=10  OutMin=0  OutMax=4  OutDataTypeStr=int8
  Cyber : Subsystem
  M : Memory
  M1 : Memory
  M3 : Memory
  Physical : Subsystem
  S1 : Subsystem
  S2 : Subsystem
  S4 : Subsystem
  W1Pos : Outport
  W2Pos : Outport  Port=2
  W4Pos : Outport  Port=3
  wires:
  Cyber/3(W4) -> Physical/3(InW4)
  Physical/3(W4) -> S4/1(PhyMeasure), W4Pos/1
  P3W4/1 -> Cyber/6(P3W4)
  S2/1(SensorOut) -> M1/1
  Physical/2(W2) -> S2/1(PhyMeasure), W2Pos/1
  DW1/1 -> Cyber/4(DW1)
  M/1 -> Cyber/1(PosW1)
  M1/1 -> Cyber/2(PosW2)
  S4/1(SensorOut) -> M3/1
  CW1C/1 -> Cyber/11(CW1C)
  P1W2/1 -> Cyber/5(P1W2)
  Cyber/2(W2) -> Physical/2(InW2)
  Cyber/1(W1) -> Physical/1(InW1)
  O1/1 -> Cyber/7(OW1)
  LD/1 -> Cyber/10(LD)
  O2/1 -> Cyber/8(OW2)
  O4/1 -> Cyber/9(OW4)
  Physical/1(W1) -> S1/1(PhyMeasure), W1Pos/1
  CW4C/1 -> Cyber/13(CW4C)
  CW2C/1 -> Cyber/12(CW2C)
  S1/1(SensorOut) -> M/1
  M3/1 -> Cyber/3(PosW4)

== system c00019M_harness/M104 ==
  DW1 : Inport  OutMin=0  OutMax=4  OutDataTypeStr=int8
  P1W2 : Inport  Port=2  OutMin=0  OutMax=4  OutDataTypeStr=int8
  P3W4 : Inport  Port=3  OutMin=0  OutMax=4  OutDataTypeStr=int8
  O1 : Inport  Port=4  OutDataTypeStr=boolean
  O2 : Inport  Port=5  OutDataTypeStr=boolean
  O4 : Inport  Port=6  OutDataTypeStr=boolean
  LD : Inport  Port=7  OutDataTypeStr=boolean
  CW1C : Inport  Port=8  OutMin=0  OutMax=4  OutDataTypeStr=int8
  CW2C : Inport  Port=9  OutMin=0  OutMax=4  OutDataTypeStr=int8
  CW4C : Inport  Port=10  OutMin=0  OutMax=4  OutDataTypeStr=int8
  Cyber : Subsystem
  M : Memory
  M1 : Memory
  M3 : Memory
  Physical : Subsystem
  S1 : Subsystem
  S2 : Subsystem
  S4 : Subsystem
  W1Pos : Outport
  W2Pos : Outport  Port=2
  W4Pos : Outport  Port=3
  wires:
  Cyber/3(W4) -> Physical/3(InW4)
  Physical/3(W4) -> S4/1(PhyMeasure), W4Pos/1
  P3W4/1 -> Cyber/6(P3W4)
  S2/1(SensorOut) -> M1/1
  Physical/2(W2) -> S2/1(PhyMeasure), W2Pos/1
  DW1/1 -> Cyber/4(DW1)
  M/1 -> Cyber/1(PosW1)
  M1/1 -> Cyber/2(PosW2)
  S4/1(SensorOut) -> M3/1
  CW1C/1 -> Cyber/11(CW1C)
  P1W2/1 -> Cyber/5(P1W2)
  Cyber/2(W2) -> Physical/2(InW2)
  Cyber/1(W1) -> Physical/1(InW1)
  O1/1 -> Cyber/7(OW1)
  LD/1 -> Cyber/10(LD)
  O2/1 -> Cyber/8(OW2)
  O4/1 -> Cyber/9(OW4)
  Physical/1(W1) -> S1/1(PhyMeasure), W1Pos/1
  CW4C/1 -> Cyber/13(CW4C)
  CW2C/1 -> Cyber/12(CW2C)
  S1/1(SensorOut) -> M/1
  M3/1 -> Cyber/3(PosW4)

== system c00019M_harness/M106 ==
  DW1 : Inport  OutMin=0  OutMax=4  OutDataTypeStr=int8
  P1W2 : Inport  Port=2  OutMin=0  OutMax=4  OutDataTypeStr=int8
  P3W4 : Inport  Port=3  OutMin=0  OutMax=4  OutDataTypeStr=int8
  O1 : Inport  Port=4  OutDataTypeStr=boolean
  O2 : Inport  Port=5  OutDataTypeStr=boolean
  O4 : Inport  Port=6  OutDataTypeStr=boolean
  LD : Inport  Port=7  OutDataTypeStr=boolean
  CW1C : Inport  Port=8  OutMin=0  OutMax=4  OutDataTypeStr=int8
  CW2C : Inport  Port=9  OutMin=0  OutMax=4  OutDataTypeStr=int8
  CW4C : Inport  Port=10  OutMin=0  OutMax=4  OutDataTypeStr=int8
  Cyber : Subsystem
  M : Memory
  M1 : Memory
  M3 : Memory
  Physical : Subsystem
  S1 : Subsystem
  S2 : Subsystem
  S4 : Subsystem
  W1Pos : Outport
  W2Pos : Outport  Port=2
  W4Pos : Outport  Port=3
  wires:
  Cyber/3(W4) -> Physical/3(InW4)
  Physical/3(W4) -> S4/1(PhyMeasure), W4Pos/1
  P3W4/1 -> Cyber/6(P3W4)
  S2/1(SensorOut) -> M1/1
  Physical/2(W2) -> S2/1(PhyMeasure), W2Pos/1
  DW1/1 -> Cyber/4(DW1)
  M/1 -> Cyber/1(PosW1)
  M1/1 -> Cyber/2(PosW2)
  S4/1(SensorOut) -> M3/1
  CW1C/1 -> Cyber/11(CW1C)
  P1W2/1 -> Cyber/5(P1W2)
  Cyber/2(W2) -> Physical/2(InW2)
  Cyber/1(W1) -> Physical/1(InW1)
  O1/1 -> Cyber/7(OW1)
  LD/1 -> Cyber/10(LD)
  O2/1 -> Cyber/8(OW2)
  O4/1 -> Cyber/9(OW4)
  Physical/1(W1) -> S1/1(PhyMeasure), W1Pos/1
  CW4C/1 -> Cyber/13(CW4C)
  CW2C/1 -> Cyber/12(CW2C)
  S1/1(SensorOut) -> M/1
  M3/1 -> Cyber/3(PosW4)

== system c00019M_harness/M107 ==
  DW1 : Inport  OutMin=0  OutMax=4  OutDataTypeStr=int8
  P1W2 : Inport  Port=2  OutMin=0  OutMax=4  OutDataTypeStr=int8
  P3W4 : Inport  Port=3  OutMin=0  OutMax=4  OutDataTypeStr=int8
  O1 : Inport  Port=4  OutDataTypeStr=boolean
  O2 : Inport  Port=5  OutDataTypeStr=boolean
  O4 : Inport  Port=6  OutDataTypeStr=boolean
  LD : Inport  Port=7  OutDataTypeStr=boolean
  CW1C : Inport  Port=8  OutMin=0  OutMax=4  OutDataTypeStr=int8
  CW2C : Inport  Port=9  OutMin=0  OutMax=4  OutDataTypeStr=int8
  CW4C : Inport  Port=10  OutMin=0  OutMax=4  OutDataTypeStr=int8
  Cyber : Subsystem
  M : Memory
  M1 : Memory
  M3 : Memory
  Physical : Subsystem
  S1 : Subsystem
  S2 : Subsystem
  S4 : Subsystem
  W1Pos : Outport
  W2Pos : Outport  Port=2
  W4Pos : Outport  Port=3
  wires:
  Cyber/3(W4) -> Physical/3(InW4)
  Physical/3(W4) -> S4/1(PhyMeasure), W4Pos/1
  P3W4/1 -> Cyber/6(P3W4)
  S2/1(SensorOut) -> M1/1
  Physical/2(W2) -> S2/1(PhyMeasure), W2Pos/1
  DW1/1 -> Cyber/4(DW1)
  M/1 -> Cyber/1(PosW1)
  M1/1 -> Cyber/2(PosW2)
  S4/1(SensorOut) -> M3/1
  CW1C/1 -> Cyber/11(CW1C)
  P1W2/1 -> Cyber/5(P1W2)
  Cyber/2(W2) -> Physical/2(InW2)
  Cyber/1(W1) -> Physical/1(InW1)
  O1/1 -> Cyber/7(OW1)
  LD/1 -> Cyber/10(LD)
  O2/1 -> Cyber/8(OW2)
  O4/1 -> Cyber/9(OW4)
  Physical/1(W1) -> S1/1(PhyMeasure), W1Pos/1
  CW4C/1 -> Cyber/13(CW4C)
  CW2C/1 -> Cyber/12(CW2C)
  S1/1(SensorOut) -> M/1
  M3/1 -> Cyber/3(PosW4)
